simulink model "Sistema1"  (R2020a)
settings: Solver=FixedStepAuto  StartTime=0.0  StopTime=10.0  FixedStep=1  RelTol=1e-3
settings Model: Creator=Miguel Gutierrez  LastModifiedBy=Miguel Gutierrez

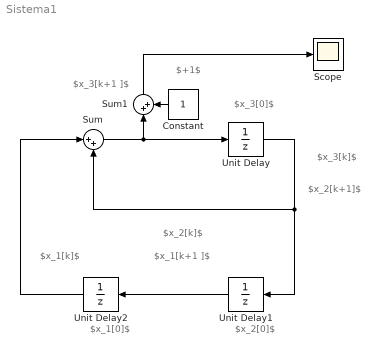
== system Sistema1 ==
  note: $x_3[k]$
  note: $x_3[k+1 ]$
  note: $x_3[0]$
  note: $x_1[k+1 ]$
  note: $x_1[0]$
  note: $x_2[k+1]$
  note: $x_2[k]$
  note: $x_1[k]$
  note: $x_2[0]$
  note: $+1$
  Constant : Constant
  Scope : Scope
  Sum : Sum  Inputs=|++
  Sum1 : Sum  Inputs=|++
  Unit Delay : UnitDelay  SampleTime=-1  HasFrameUpgradeWarning=on
  Unit Delay1 : UnitDelay  InitialCondition=1  SampleTime=-1  HasFrameUpgradeWarning=on
  Unit Delay2 : UnitDelay  InitialCondition=1  SampleTime=-1  HasFrameUpgradeWarning=on
  wires:
  Unit Delay/1 -> Sum/2, Unit Delay1/1
  Unit Delay1/1 -> Unit Delay2/1
  Unit Delay2/1 -> Sum/1
  Constant/1 -> Sum1/2
  Sum/1 -> Sum1/1, Unit Delay/1
  Sum1/1 -> Scope/1
